simulink model "OneWheelModel"  (R2021b)
settings: Solver=ode4  StartTime=0.0  StopTime=1  FixedStep=0.001  RelTol=1e-3
values from neighbouring files (symbols this model uses):
  afx_f = [1.736519934348130,-2.903281841026900e-04,2.651682004580759,7.000047010028531e+04,3.270011055825476e+03,-0.001252141095807,1.596836353939939]    [OneWheelModel_test1.m]    (also in OneWheelModel_test2.m)
  Iwf = 0.2    [OneWheelModel_test1.m]    (also in OneWheelModel_test2.m)
  M = 260    [OneWheelModel_test1.m]    (also in OneWheelModel_test2.m)
  mu_tire_F = 0.55    [OneWheelModel_test1.m]    (also in OneWheelModel_test2.m)
  Rwf = 18*(25.4/1000)/2    (= 0.2286)    [OneWheelModel_test1.m]    (also in OneWheelModel_test2.m)
undefined symbols (not defined in the file or in its folder): g, gear_f, Mwf, W0_R
libraries: simulink x1
settings Model: Creator=tsuyoshi  LastModifiedBy=tsuyoshi

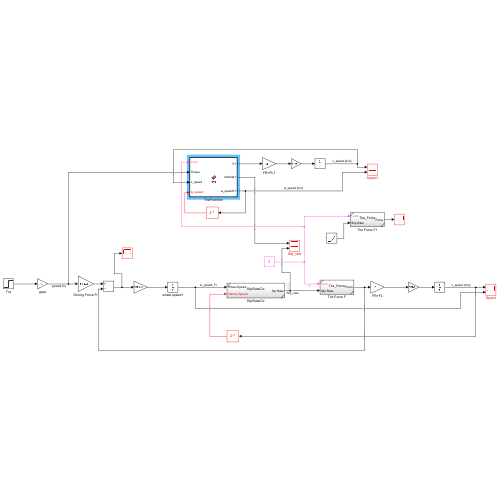
[thumbnail: Simulink's stored preview of the top-level diagram]
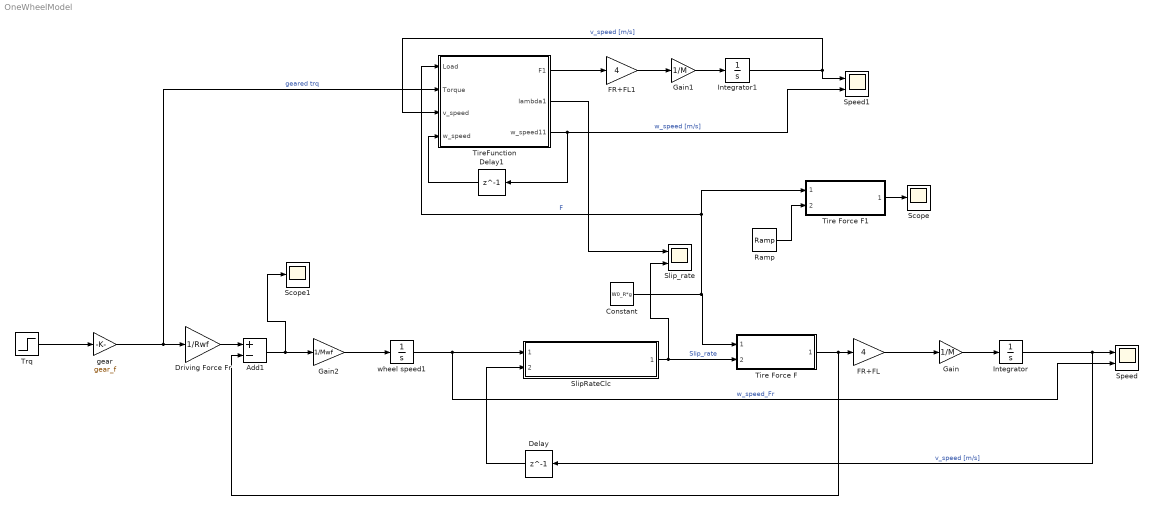
== system OneWheelModel ==
  Add1 : Sum  Inputs=+-
  Constant : Constant  Value=W0_R*g
  Delay : Delay  DelayLength=1
  Delay1 : Delay  DelayLength=1
  Driving Force Fr : Gain  Gain=1/Rwf
  FR+FL : Gain  Gain=4
  FR+FL1 : Gain  Gain=4
  Gain : Gain  Gain=1/M
  Gain1 : Gain  Gain=1/M
  Gain2 : Gain  Gain=1/Mwf
  Integrator : Integrator
  Integrator1 : Integrator
  Ramp : simulink/Sources/Ramp  slope=0.1  start=0  InitialOutput=0
  Scope : Scope
  Scope1 : Scope
  SlipRateClc : Subsystem  ReferencedSubsystem=SlipRateClc
  Slip_rate : Scope  NumInputPorts=2
  Speed : Scope  NumInputPorts=2
  Speed1 : Scope  NumInputPorts=2
  Tire Force F : Subsystem  ReferencedSubsystem=Tire_Force
  Tire Force F1 : Subsystem  ReferencedSubsystem=Tire_Force
  TireFunction : MATLAB Function  TreatAsAtomicUnit=on
  Trq : Step  Time=0.2  After=5  SampleTime=0
  gear : Gain  Gain=gear_f
  wheel speed1 : Integrator  LowerSaturationLimit=0
  wires:
  SlipRateClc/1 -> Slip_rate/2, Tire Force F/2  "Slip_rate"
  Driving Force Fr/1 -> Add1/1
  Constant/1 -> TireFunction/1(Load), Tire Force F1/1, Tire Force F/1  "F"
  Integrator/1 -> Speed/1, Delay/1  "v_speed [m/s]"
  Tire Force F/1 -> FR+FL/1, Add1/2
  wheel speed1/1 -> Speed/2, SlipRateClc/1  "w_speed_Fr"
  Gain/1 -> Integrator/1
  Trq/1 -> gear/1
  gear/1 -> TireFunction/2(Torque), Driving Force Fr/1  "geared trq"
  FR+FL/1 -> Gain/1
  Ramp/1 -> Tire Force F1/2
  Tire Force F1/1 -> Scope/1
  Gain2/1 -> wheel speed1/1
  Add1/1 -> Gain2/1, Scope1/1
  Delay/1 -> SlipRateClc/2
  FR+FL1/1 -> Gain1/1
  Gain1/1 -> Integrator1/1
  TireFunction/3(w_speed11) -> Delay1/1, Speed1/2  "w_speed [m/s]"
  Integrator1/1 -> Speed1/1, TireFunction/3(v_speed)  "v_speed [m/s]"
  TireFunction/1(F1) -> FR+FL1/1
  Delay1/1 -> TireFunction/4(w_speed)
  TireFunction/2(lambda1) -> Slip_rate/1

== matlab function OneWheelModel/TireFunction ==
  data: Load input; Torque input; v_speed input; F1 output; w_speed input; Rwf parameter; Iwf parameter; afx_f parameter; mu_tire_F parameter; lambda1 output; w_speed11 output
function [F1,lambda1,w_speed11] = fcn(Load, Torque, v_speed, w_speed, Rwf, Iwf, afx_f, mu_tire_F)
%%
% Input
% v_speed : vehicle speed [m/s]
% w_speed : wheel speed [m/s]

%% main
if w_speed==0
    if Torque>0
        F1=0;
        lambda1=1;
        w_speed11=100;
    else
        F1=0;
        lambda1=0;
        w_speed11=0;
    end
else
    timestep=0.001;
    x0=0.1;
    options=optimoptions('fsolve','Algorithm','Levenberg-Marquardt');
    w_speed_dot = fsolve(@myfun,x0,options);
    
    w_speed11=w_speed + w_speed_dot*timestep;
    lambda1=(w_speed11-v_speed)/w_speed11;
    C1 = afx_f(1);
    D1 = (Load*afx_f(2) + afx_f(3))*Load;
    E1 = Load*afx_f(6) + afx_f(7);
    B1 = afx_f(4)*sin(2*atan(Load/afx_f(5)))/(D1*C1);
    F1 = D1*sin(C1*atan(B1*lambda1-E1*(B1*lambda1-atan(B1*lambda1))))*mu_tire_F;
end  

    function Error=myfun(w_speed_dot)
        w_speed1=w_speed + w_speed_dot*timestep;
        lambda=(w_speed1-v_speed)/w_speed1;
        C = afx_f(1);
        D = (Load*afx_f(2) + afx_f(3))*Load;
        E = Load*afx_f(6) + afx_f(7);
        B = afx_f(4)*sin(2*atan(Load/afx_f(5)))/(D*C);
        F = D*sin(C*atan(B*lambda-E*(B*lambda-atan(B*lambda))))*mu_tire_F;
        Error = Iwf*w_speed_dot/Rwf + Rwf*F - Torque;
    end
end



% function lambda=SlipRate(w_speed, v_speed)
%     lambda=(w_speed-v_speed)/w_speed;
% %     lambda=(w_speed-v_speed)/max(w_speed,v_speed,eps);
% %     if lambda>1 
% %         lambda=1;
% %     elseif lambda<0
% %         lambda=0;
% %     end
% end
